simulink model "SSRP_A"  (R2023a)
settings: Solver=FixedStepAuto  StartTime=0.0  StopTime=inf  RelTol=1e-3
libraries: androidsensorlib x5, androiduilib x5, androidcommunicationlib x3, androidaudiovideolib x2
settings Model: Creator=parag  LastModifiedBy=parag
settings OptimizationCC: EnhancedBackFolding=on  PassReuseOutputArgsAs=Individual arguments  ZeroExternalMemoryAtStartup=off  ZeroInternalMemoryAtStartup=off  MaxStackSize=64  OptimizeBlockOrder=speed  DifferentSizesBufferReuse=on  OptimizationCustomize=off  EfficientTunableParamExpr=on
settings DebuggingCC: ParameterTunabilityLossMsg=error
settings HardwareCC: ProdBitPerPointer=32  ProdBitPerSizeT=32  ProdBitPerPtrDiffT=32  ProdLargestAtomicInteger=Long  ProdLargestAtomicFloat=Double  ProdWordSize=32  ProdHWDeviceType=ARM Compatible->ARM Cortex  UseEmbeddedCoderFeatures=off  UseSimulinkCoderFeatures=off
settings SFSimCC: MATLABDynamicMemAlloc=off
settings RTWCC: Description=Embedded Coder  SystemTargetFile=ert.tlc  HardwareBoard=Android Device  TLCOptions="-aInlineSetEventsForThisBaseRateFcn=TLC_FALSE -aSuppressMultiTaskScheduler=TLC_FALSE  -aRateBasedStepFcn=0"  TemplateMakefile=ert_default_tmf  RTWVerbose=off  Toolchain=Android SDK/NDK Tools
settings CodeAppCC: ForceParamTrailComments=on  IgnoreCustomStorageClasses=off  OperatorAnnotations=on  SimulinkDataObjDesc=on  SFDataObjDesc=on  InsertBlockDesc=on
settings ERTTargetCC: SupportNonInlinedSFcns=on

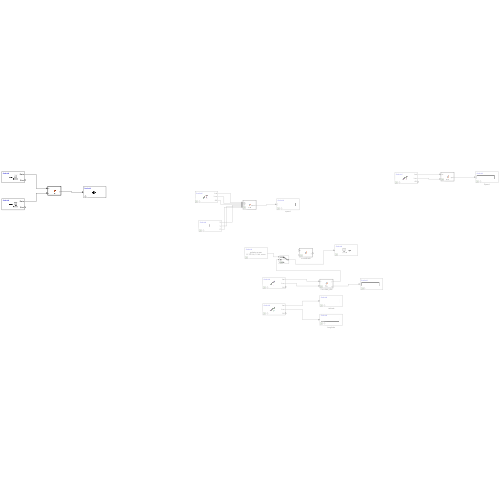
[thumbnail: Simulink's stored preview of the top-level diagram]
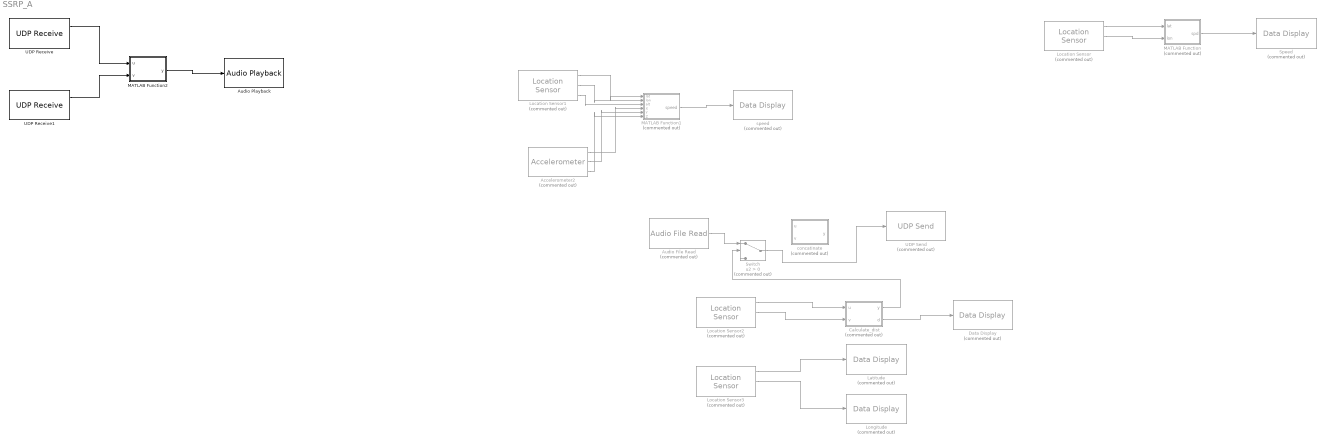
== system SSRP_A ==
  Accelerometer2 : androidsensorlib/Accelerometer  Commented=on  OutputVector=off  SampleTime=0.1  BlockPlatform=Android
  Audio File Read : androidaudiovideolib/Audio File Read  Commented=on  FileName=guitartune.wav  FrameSize=4410
  Audio Playback : androidaudiovideolib/Audio Playback  SampleFreq=44100  AudioSamplingFreq=44100  SampleTime=0.1  DeviceStr=0  QueueDuration=0  BlockPlatform=Android
  Calculate_dist : MATLAB Function  Commented=on  TreatAsAtomicUnit=on
  Data Display : androiduilib/Data Display  Commented=on  DataDisplayId=SSRP_A/Data_Display  Format=Float  Precision=6  SimulateUsing=Code generation  blockPlatform=Android
  Latitude : androiduilib/Data Display  Commented=on  DataDisplayId=SSRP_A/Latitude  Format=Float  Precision=6  SimulateUsing=Code generation  blockPlatform=Android
  Location Sensor{,1..3} (4 alike) : androidsensorlib/Location Sensor  Commented=on  OutputVector=off  SampleTime=0.1  BlockPlatform=Android
  Longitude : androiduilib/Data Display  Commented=on  DataDisplayId=SSRP_A/Longitude  Format=Float  Precision=6  SimulateUsing=Code generation  blockPlatform=Android
  MATLAB Function : MATLAB Function  Commented=on  TreatAsAtomicUnit=on
  MATLAB Function1 : MATLAB Function  Commented=on  TreatAsAtomicUnit=on
  MATLAB Function2 : MATLAB Function  TreatAsAtomicUnit=on
  Speed : androiduilib/Data Display  Commented=on  DataDisplayId=SSRP_A/Speed  Format=Float  Precision=6  SimulateUsing=Code generation  blockPlatform=Android
  Switch : Switch  Commented=on  Criteria=u2 > Threshold  SaturateOnIntegerOverflow=off  InputSameDT=off
  UDP Receive : androidcommunicationlib/UDP Receive  localURL='0.0.0.0'  localPort=26004  remoteURL='0.0.0.0'  remotePort=-1  recvBufferSize=8192  signalDatatype=int16  dims=4410  isVarSize=off  showBlockingTime=off  blockingTime=0  sampletime=0.1  blockPlatform=Android
  UDP Receive1 : androidcommunicationlib/UDP Receive  localURL='0.0.0.0'  localPort=26004  remoteURL='0.0.0.0'  remotePort=-1  recvBufferSize=8192  signalDatatype=int16  dims=4410  isVarSize=off  showBlockingTime=off  blockingTime=0  sampletime=0.1  blockPlatform=Android
  UDP Send : androidcommunicationlib/UDP Send  Commented=on  remoteURL='255.255.255.255'  remotePort=25000  localURL='0.0.0.0'  localPortSource=Automatically determine  localPort=-1  sampletime=-1  blockPlatform=Android  separateLengthPort=0
  concatinate : MATLAB Function  Commented=on  TreatAsAtomicUnit=on
  speed : androiduilib/Data Display  Commented=on  DataDisplayId=SSRP_A/speed  Format=Float  Precision=6  SimulateUsing=Code generation  blockPlatform=Android
  wires:
  Location Sensor/1 -> MATLAB Function/1(lat)
  Location Sensor/2 -> MATLAB Function/2(lon)
  MATLAB Function/1(spd) -> Speed/1
  Location Sensor1/1 -> MATLAB Function1/1(lat)
  Location Sensor1/2 -> MATLAB Function1/2(lon)
  Location Sensor1/3 -> MATLAB Function1/3(alt)
  Accelerometer2/1 -> MATLAB Function1/4(X)
  Accelerometer2/2 -> MATLAB Function1/5(Y)
  Accelerometer2/3 -> MATLAB Function1/6(Z)
  MATLAB Function1/1(speed) -> speed/1
  Location Sensor2/1 -> Calculate_dist/1(u)
  Location Sensor2/2 -> Calculate_dist/2(v)
  Calculate_dist/2(d) -> Data Display/1
  Location Sensor3/1 -> Latitude/1
  Location Sensor3/2 -> Longitude/1
  Audio File Read/1 -> Switch/1
  Calculate_dist/1(y) -> Switch/2
  Switch/1 -> UDP Send/1
  UDP Receive/1 -> MATLAB Function2/1(u)
  UDP Receive1/1 -> MATLAB Function2/2(v)
  MATLAB Function2/1(y) -> Audio Playback/1

== matlab function SSRP_A/MATLAB Function1 ==
  data: lat input; speed output; lon input; alt input; X input; Y input; Z input
function speed = fcn(lat, lon, alt, X, Y, Z)
    % Initialize the Kalman filter parameters
    A = eye(6); % State transition matrix
    B = [0; 0; 0; 0; 0; -9.81]; % Control input matrix
    H = [0 0 0 1 0 0; 0 0 0 0 1 0; 0 0 0 0 0 1]; % Measurement matrix

    % Initialize the state estimate and covariance matrix
    x_hat = zeros(6, 1); % Initial state estimate
    P = eye(6); % Initial covariance matrix

    % Loop for real-time updates
    while true
        % Get accelerometer readings and GPS data in real-time
        accelerometer_x = X; % X-axis accelerometer reading
        accelerometer_y = Y; % Y-axis accelerometer reading
        accelerometer_z = Z; % Z-axis accelerometer reading
        latitude = lat; % GPS latitude
        longitude = lon; % GPS longitude
        altitude = alt; % GPS altitude

        % Perform Kalman filter prediction step
        x_hat_minus = A * x_hat + B * [accelerometer_x; accelerometer_y; accelerometer_z];
        P_minus = A * P * A';

        % Perform Kalman filter update step
        z = [latitude; longitude; altitude];
        R = eye(3); % Measurement noise covariance matrix
        K = P_minus * H' / (H * P_minus * H' + R);
        x_hat = x_hat_minus + K * (z - H * x_hat_minus);
        P = (eye(size(A)) - K * H) * P_minus;

        % Calculate speed from the estimated velocity components
        speed = norm(x_hat(4:6));

        % Use the updated state estimate for speed estimation or any other purpose
        % ...

        % Pause or sleep for a desired time interval before the next update
        pause(0.1); % Adjust the time interval as per your requirements
    end
end

== matlab function SSRP_A/MATLAB Function ==
  data: lat input; spd output; lon input
function spd = fcn(lat, lon)
   l = length(lat);
   radius= 6371.00;
   time =1;
   spd =zeros(l,1);
   for t= 1:l
       if t>1
           oldLat = lat(t);
           oldlon = lon(t);
           newLat = lat(t-1);
           newLon = lon(t-1);
           dLat = deg2rad(newLat-oldLat);
           dLon = deg2rad(newLon- oldlon);
           a = sin(dLat/2) * sin(dLat/2) +  ...
               cos(deg2rad(oldLat)) *cos(deg2rad(newLat)) * ...
               sin(dLon/2) * sin(dLon/2);
           c = 2 * asin(sqrt(a));
           spd(t) =  (6371.00 * c*1609.00 *60)/1000;
       else
           spd(t) = 0;
       end
   end

== matlab function SSRP_A/concatinate ==
  data: u input; y output; v input
function y = fcn(u,v)
    if v == 0
        y = u ;
    else 
        y = zeros(4410, 1,'int16');
end; 

endfunction y = fcn(u)

y = u;

== matlab function SSRP_A/Calculate_dist ==
  data: u input; y output; v input; d output
function [y,d] = fcn(u, v)
N = 4410;
freq = 600;

% Calculate the sampling frequency needed for a 10-second duration
duration = 10;  % Duration in seconds
Fs = N / duration;

% Generate a time vector
t = (0:N-1) / Fs;

% Generate the sine wave
sound_array = zeros(N, 2, 'int16');
khali = zeros(N, 2, 'int16');
%starts N x 2 matrix
sound_array(:,1) = int16(sin(2*pi*freq*t));
sound_array(:,2) = int16(sin(2*pi*freq*t));

% Define the center of the circle
center_lat = 23.210336;  % Latitude of the center
center_lon = 72.683842;  % Longitude of the center

% Define the radius of the circle (you need to set this value)
radius_km = 0.08;  % Replace with the desired radius in kilometers

% Earth's mean radius in kilometers
earth_radius_km = 6371;

% Convert latitude and longitude from degrees to radians
center_lat_rad = deg2rad(center_lat);
center_lon_rad = deg2rad(center_lon);
point_lat_rad = deg2rad(u);
point_lon_rad = deg2rad(v);

% Calculate the Haversine distance between the center and the point
dlat = point_lat_rad - center_lat_rad;
dlon = point_lon_rad - center_lon_rad;

a = sin(dlat/2)^2 + cos(center_lat_rad) * cos(point_lat_rad) * sin(dlon/2)^2;
c = 2 * atan2(sqrt(a), sqrt(1 - a));
distance_km = earth_radius_km * c;
d = distance_km  ;
% Check if the point is inside the circle
if distance_km <= radius_km
    y = 1;
else
    y = 0;
end
end

== matlab function SSRP_A/MATLAB Function2 ==
  data: u input; y output; v input
function y = fcn(u,v)    
        y = [u,v];
end
